simulink library "tqd"  (R2021b)
settings: Solver=VariableStepAuto  StartTime=0.0  StopTime=10.0  RelTol=1e-3
undefined symbols (not defined in the file or in its folder): ATQD_BOSEnBPSPosn_X_kph, ATQD_BOSMap_X_rpm, ATQD_BOSMap_Y_pct, ATQD_CreepBaseTqD_X_kph, ATQD_CreepBaseTqD_Y_Deg, ATQD_CreepBaseTqR_X_kph, ATQD_CreepBaseTqR_Y_Deg, ATQD_CreepBPSDisPosn_X_Deg, ATQD_CreepBPSDisPosnR_X_Deg, ATQD_CreepBPSEnPosn_X_Deg, ATQD_CreepBPSEnPosnR_X_Deg, ATQD_CreepDeltaTq_X_kph, ATQD_CreepIterm_X_kph, ATQD_CreepIterm_Y_kph, ATQD_CreepItermMaxLimit_X_pct, ATQD_CreepPreloadTime_X_kph, ATQD_CreepPreloadTq_X_kph, ATQD_CreepPreloadTq_Y_s, ATQD_CreepProtTq_X_Deg, ATQD_CreepPterm_X_kph, ATQD_ECOTqMapD_X_rpm, ATQD_ECOTqMapD_Y_pct, ATQD_NL1TqMapD_X_rpm, ATQD_NL1TqMapD_Y_pct, ATQD_NRMRrEDUSpRat_X_rpm, ATQD_NRMRrEDUSpRat_Y_Nm, ATQD_PedalMapClimbUpLim_X_rpm, ATQD_PedalMapClimbUpLim_Y_Deg, ATQD_PreLoadTq_X_s, ATQD_SL1TqMapD_X_rpm, ATQD_SL1TqMapD_Y_pct, ATQD_WhlTqCapMotGain_X_pct, ATQD_WhlTqCapMotGain_Y_mV, ENUM_ACCPEDALLOWSW_LOWIDLE, ENUM_ACCPEDALLOWSW_NOIDLE, ENUM_CHRGPLUGSTA_NONE, ENUM_CRASHSTATE_NOCRASH, ENUM_DCDCFAULTSTA_WORKING, ENUM_DRIVEMODE_ECO, ENUM_DRIVEMODE_NRM, ENUM_DRIVEMODE_SPORT, ENUM_DRIVETRAIN_AWD, ENUM_DRIVETRAIN_FWD, ENUM_DRIVETRAIN_RWD, ENUM_EBSBRKSW_PRESSED, ENUM_EBSTORQUERWQ_LIMIT, ENUM_EBSTORQUERWQ_TORQUE, ENUM_EMTRQMODE_ACCL, ENUM_EMTRQMODE_BRAKING, ENUM_EMTRQMODE_COASTING, ENUM_EPBERROR_NORMAL, ENUM_EPBSTA_APPLIED, ENUM_EPBSTA_RELEASED, ENUM_EPBSTA_UNKNOWN, ENUM_EPBSTARAW_NOTSET, ENUM_EPBSTARAW_SET, ENUM_GEARACTUALPOSN_D, ENUM_GEARACTUALPOSN_N, ENUM_GEARACTUALPOSN_P, ENUM_GEARACTUALPOSN_R ... (+201)
libraries: hcu_lib x19, simulink x12
(part 6 of 6)

== system tqd/TQD/TorqueDemand/TorqueModule/DriverWhlTqDem/RollingRegenJudge ==
  VDHP_LowIdleAccPedal_flg : Inport
  VINP_VehSpd_kph : Inport  Port=2
  VTQD_TqTargetShaftSpd_rpm : Inport  Port=3
  VTQD_RollRegenDisableReq_flg : Inport  Port=4
  VTQD_TqSourceFr_enum : Inport  Port=5
  VTQD_TqSourceRr_enum : Inport  Port=6
  VTQD_CreepEnable_flg : Inport  Port=7
  Constant : Constant  Value=ENUM_TQSOURCE_CC
  Constant1 : Constant  Value=ENUM_TQSOURCE_ADAS
  Constant2 : Constant  Value=ENUM_TQSOURCE_APS
  Constant3 : Constant  Value=ENUM_TQSOURCE_CC
  Constant4 : Constant  Value=ENUM_TQSOURCE_ADAS
  Constant5 : Constant  Value=ENUM_TQSOURCE_APS
  Detect Increase : simulink/Logic and Bit Operations/Detect Increase  vinit=0.0  OutDataTypeStr=boolean
  Equal{,1..5} (6 alike) : RelationalOperator  Operator===  OutDataTypeStr=boolean  RndMeth=Simplest
  Logical Operator : Logic  Inputs=5  AllPortsSameDT=off  OutDataTypeStr=boolean
  Logical Operator1 : Logic  Operator=NOT  AllPortsSameDT=off  OutDataTypeStr=boolean
  Logical Operator10 : Logic  Operator=OR  AllPortsSameDT=off  OutDataTypeStr=boolean
  Logical Operator11 : Logic  Operator=NOT  AllPortsSameDT=off  OutDataTypeStr=boolean
  Logical Operator12 : Logic  Operator=NOT  AllPortsSameDT=off  OutDataTypeStr=boolean
  Logical Operator5 : Logic  Operator=OR  Inputs=3  AllPortsSameDT=off  OutDataTypeStr=boolean
  Logical Operator9 : Logic  Operator=OR  Inputs=3  AllPortsSameDT=off  OutDataTypeStr=boolean
  Relay : Relay  OnSwitchValue=KTQD_RegenOnSpd_kph  OffSwitchValue=KTQD_RegenOffSpd_kph
      settings: AttributesFormatString=|
      | ON: %<OnSwitchValue>
      | OFF: %<OffSwitchValue>
  Switch2 : Switch  Criteria=u2 ~= 0
      settings: AttributesFormatString=<%<Criteria>>
  Unit Delay : UnitDelay  SampleTime=-1  HasFrameUpgradeWarning=on
  Unit Delay1 : UnitDelay  SampleTime=-1  HasFrameUpgradeWarning=on
  VTQD_RollRegenEnable_flg : Outport
  VTQD_RollingShaftSpd_rpm : Outport  Port=2
  wires:
  Equal5/1 -> Logical Operator9/3
  Equal3/1 -> Logical Operator9/1
  Equal4/1 -> Logical Operator9/2
  Constant4/1 -> Equal4/2
  [VTQD_TqSourceRr_enum] -> Equal4/1
  Constant5/1 -> Equal5/2
  [VTQD_TqSourceRr_enum] -> Equal5/1
  Constant3/1 -> Equal3/2
  [VTQD_TqSourceRr_enum] -> Equal3/1
  Constant2/1 -> Equal2/2
  [VTQD_TqSourceFr_enum] -> Equal2/1
  Constant1/1 -> Equal1/2
  [VTQD_TqSourceFr_enum] -> Equal1/1
  Constant/1 -> Equal/2
  Logical Operator11/1 -> Logical Operator/5
  Logical Operator10/1 -> Logical Operator11/1
  Logical Operator9/1 -> Logical Operator10/2
  Logical Operator5/1 -> Logical Operator10/1
  [VTQD_CreepEnable_flg] -> Unit Delay1/1
  Equal2/1 -> Logical Operator5/3
  Equal1/1 -> Logical Operator5/2
  Equal/1 -> Logical Operator5/1
  VTQD_CreepEnable_flg/1 -> [VTQD_CreepEnable_flg]
  VTQD_TqSourceFr_enum/1 -> [VTQD_TqSourceFr_enum]
  VTQD_TqSourceRr_enum/1 -> [VTQD_TqSourceRr_enum]
  [VTQD_RollRegenDisableReq_flg] -> Logical Operator1/1
  VTQD_RollRegenDisableReq_flg/1 -> [VTQD_RollRegenDisableReq_flg]
  Unit Delay/1 -> Switch2/3
  Switch2/1 -> VTQD_RollingShaftSpd_rpm/1, Unit Delay/1  "VTQD_RollingShaftSpd_rpm"
  [VTQD_TqTargetShaftSpd_rpm] -> Switch2/1
  Detect Increase/1 -> Switch2/2
  [VTQD_RollRegenEnable_flg] -> Detect Increase/1
  VTQD_TqTargetShaftSpd_rpm/1 -> [VTQD_TqTargetShaftSpd_rpm]
  [VINP_VehSpd_kph] -> Relay/1
  VINP_VehSpd_kph/1 -> [VINP_VehSpd_kph]
  VDHP_LowIdleAccPedal_flg/1 -> [VTQD_LowIdleAccPedal_flg]
  Logical Operator/1 -> VTQD_RollRegenEnable_flg/1, [VTQD_RollRegenEnable_flg]  "VTQD_RollRegenEnable_flg"
  Unit Delay1/1 -> Logical Operator12/1
  Relay/1 -> Logical Operator/2
  Logical Operator12/1 -> Logical Operator/4
  Logical Operator1/1 -> Logical Operator/3
  [VTQD_LowIdleAccPedal_flg] -> Logical Operator/1
  [VTQD_TqSourceFr_enum] -> Equal/1

== system tqd/TQD/TorqueDemand/TorqueModule/TqCoordination/Coordinate_DirverPedal ==
  VTQD_DriverWhlTqDem_Nm : Inport
  Action Port : ActionPort
  Constant9 : Constant  Value=ENUM_TQSOURCE_INTERNAL
  VTQD_DriverWhlTqReq_Nm : Outport
  VTQD_TqSourceInternal_enum : Outport  Port=2
  wires:
  VTQD_DriverWhlTqDem_Nm/1 -> VTQD_DriverWhlTqReq_Nm/1
  Constant9/1 -> VTQD_TqSourceInternal_enum/1

== system tqd/TQD/TorqueDemand/TorqueModule/TqCoordination/Coordinate_NoSuitbleGear_flg ==
  Action Port : ActionPort
  Constant5 : Constant  Value=KTQD_DriverTqDemN_Nm
  Constant8 : Constant  Value=ENUM_TQSOURCE_INVALID
  VTQD_GearNoSuitReq_Nm : Outport
  VTQD_TqSourceGearNoSuit_enum : Outport  Port=2
  wires:
  Constant5/1 -> VTQD_GearNoSuitReq_Nm/1
  Constant8/1 -> VTQD_TqSourceGearNoSuit_enum/1

== system tqd/TQD/TorqueDemand/TorqueModule/TqDistribution/AWD_Ratio ==
  VTQD_DriverWhlTqDem_Nm : Inport
  VTQD_RrShaftSpd_rpm : Inport  Port=2
  VTQD_EVDriveMode_enum : Inport  Port=3
  VTQD_LimpHomeAct_flg : Inport  Port=4
  VTQD_CreepPrLoadEnable_flg : Inport  Port=5
  Action Port : ActionPort
  Constant : Constant  Value=ONE_FLOAT
  Constant1 : Constant  Value=ONE_FLOAT
  Constant10 : Constant  Value=KTQD_AWDRrRatio_rat_ovrdflg  VectorParams1D=off  SampleTime=-1
  Constant11 : Constant  Value=KTQD_AWDRrRatio_rat_ovrdval  VectorParams1D=off  SampleTime=-1
  Constant2 : Constant  Value=ENUM_DRIVEMODE_ECO
  Constant5 : Constant  Value=ENUM_DRIVEMODE_SPORT
  Constant8 : Constant  Value=KTQD_AWDFrRatio_rat_ovrdflg  VectorParams1D=off  SampleTime=-1
  Constant9 : Constant  Value=KTQD_AWDFrRatio_rat_ovrdval  VectorParams1D=off  SampleTime=-1
  Equal : RelationalOperator  Operator===  OutDataTypeStr=boolean  RndMeth=Simplest
  Equal2 : RelationalOperator  Operator===  OutDataTypeStr=boolean  RndMeth=Simplest
  LiuzgSwitch{1..3,13} (4 alike) : Switch  Criteria=u2 ~= 0
      settings: AttributesFormatString=<%<Criteria>>
  MTQD_ECORrEDUSpRat_Z_rat : Lookup_n-D  BreakpointsForDimension1=ATQD_NRMRrEDUSpRat_Y_Nm  BreakpointsForDimension2=ATQD_NRMRrEDUSpRat_X_rpm  Table=MTQD_ECORrEDUSpRat_Z_rat  ExtrapMethod=Clip  InternalRulePriority=Speed  RndMeth=Simplest  InputSameDT=on
      settings: InputPortMap=u0,u1
  "MTQD_NRMRrEDUSpRat_Z_rat  " : Lookup_n-D  BreakpointsForDimension1=ATQD_NRMRrEDUSpRat_Y_Nm  BreakpointsForDimension2=ATQD_NRMRrEDUSpRat_X_rpm  Table=MTQD_NRMRrEDUSpRat_Z_rat  ExtrapMethod=Clip  InternalRulePriority=Speed  RndMeth=Simplest  InputSameDT=on
      settings: InputPortMap=u0,u1
  "MTQD_SPORTRrEDUSpRat_Z_rat " : Lookup_n-D  BreakpointsForDimension1=ATQD_NRMRrEDUSpRat_Y_Nm  BreakpointsForDimension2=ATQD_NRMRrEDUSpRat_X_rpm  Table=MTQD_SPORTRrEDUSpRat_Z_rat  ExtrapMethod=Clip  InternalRulePriority=Speed  RndMeth=Simplest  InputSameDT=on
      settings: InputPortMap=u0,u1
  Saturation : Saturate  UpperLimit=KTQD_RrEDUTqDistrictMax_gain  LowerLimit=KTQD_RrEDUTqDistrictMin_gain
      settings: AttributesFormatString=|
      | <%<UpperLimit>>
      | <%<LowerLimit>>
  Subtract : Sum  Inputs=+-
  Switch : Switch  Criteria=u2 > Threshold
  Switch1 : Switch  Criteria=u2 > Threshold
  VTQD_FrRatio_AWD : Outport
  VTQD_RrRatio_AWD : Outport  Port=2
  wires:
  Constant/1 -> Subtract/1
  Saturation/1 -> Switch1/3, Subtract/2
  VTQD_EVDriveMode_enum/1 -> [VTQD_EVDriveMode_enum]
  VTQD_DriverWhlTqDem_Nm/1 -> [VTQD_DriverWhlTqDem_Nm]
  VTQD_RrShaftSpd_rpm/1 -> [VTQD_RrShaftSpd_rpm]
  [VTQD_DriverWhlTqDem_Nm] -> "MTQD_NRMRrEDUSpRat_Z_rat  "/1
  [VTQD_RrShaftSpd_rpm] -> "MTQD_NRMRrEDUSpRat_Z_rat  "/2
  VTQD_LimpHomeAct_flg/1 -> [VTQD_LimpHomeAct_flg]
  [VTQD_LimpHomeAct_flg] -> LiuzgSwitch13/2
  Equal/1 -> LiuzgSwitch1/2
  "MTQD_SPORTRrEDUSpRat_Z_rat "/1 -> LiuzgSwitch1/1
  [VTQD_EVDriveMode_enum] -> Equal/1
  Constant5/1 -> Equal/2
  [VTQD_DriverWhlTqDem_Nm] -> "MTQD_SPORTRrEDUSpRat_Z_rat "/1
  [VTQD_RrShaftSpd_rpm] -> "MTQD_SPORTRrEDUSpRat_Z_rat "/2
  "MTQD_NRMRrEDUSpRat_Z_rat  "/1 -> LiuzgSwitch1/3, LiuzgSwitch13/1
  [VTQD_RrShaftSpd_rpm] -> MTQD_ECORrEDUSpRat_Z_rat/2
  [VTQD_DriverWhlTqDem_Nm] -> MTQD_ECORrEDUSpRat_Z_rat/1
  Constant2/1 -> Equal2/2
  [VTQD_EVDriveMode_enum] -> Equal2/1
  MTQD_ECORrEDUSpRat_Z_rat/1 -> LiuzgSwitch3/1
  Equal2/1 -> LiuzgSwitch3/2
  LiuzgSwitch3/1 -> LiuzgSwitch13/3
  LiuzgSwitch1/1 -> LiuzgSwitch3/3
  [VTQD_CreepPrLoadEnable_flg] -> LiuzgSwitch2/2
  Constant1/1 -> LiuzgSwitch2/1
  VTQD_CreepPrLoadEnable_flg/1 -> [VTQD_CreepPrLoadEnable_flg]
  LiuzgSwitch13/1 -> LiuzgSwitch2/3
  Subtract/1 -> Switch/3
  Switch/1 -> VTQD_FrRatio_AWD/1  "VTQD_FrEDUSpRat_rat"
  Switch1/1 -> VTQD_RrRatio_AWD/1  "VTQD_RrEDUSpRat_rat"
  Constant8/1 -> Switch/2
  Constant9/1 -> Switch/1
  Constant11/1 -> Switch1/1
  Constant10/1 -> Switch1/2
  LiuzgSwitch2/1 -> Saturation/1

== system tqd/TQD/TorqueDemand/TorqueModule/TqDistribution/FWD_Ratio ==
  Action Port : ActionPort
  Constant : Constant  Value=ONE_FLOAT
  Constant1 : Constant  Value=ZERO_FLOAT
  VTQD_FrRatio_FWD : Outport
  VTQD_RrRatio_FWD : Outport  Port=2
  wires:
  Constant/1 -> VTQD_FrRatio_FWD/1
  Constant1/1 -> VTQD_RrRatio_FWD/1

== system tqd/TQD/TorqueDemand/TorqueModule/TqDistribution/RWD_Ratio ==
  Action Port : ActionPort
  Constant : Constant  Value=ONE_FLOAT
  Constant1 : Constant  Value=ZERO_FLOAT
  VTQD_FrRatio_RWD : Outport
  VTQD_RrRatio_RWD : Outport  Port=2
  wires:
  Constant1/1 -> VTQD_FrRatio_RWD/1
  Constant/1 -> VTQD_RrRatio_RWD/1

== system tqd/TQD/TorqueDemand/TorqueModule/AvaliableTqLimit/TorqueCapacityCalcalation/CapacityDistribution ==
  VTQD_FrEDUSpRat_cmd : Inport
  VTQD_RrEDUSpRat_rat : Inport  Port=2
  VTQD_TMPwrAvailDchrg_kW : Inport  Port=3
  VINP_HVBPwrAvailChrg_kw : Inport  Port=4
  Abs1 : Abs
  Product{,1,4..5} (4 alike) : Product
  VTQD_FrHVBPwrAvailDchrg_kw : Outport
  VTQD_RrHVBPwrAvailDchrg_kw : Outport  Port=2
  VTQD_FrHVBPwrAvailChrg_kw : Outport  Port=3
  VTQD_RrHVBPwrAvailChrg_kw : Outport  Port=4
  wires:
  VTQD_RrEDUSpRat_rat/1 -> [VTQD_RrEDUSpRat_rat]
  VTQD_FrEDUSpRat_cmd/1 -> [VTQD_FrEDUSpRat_rat]
  VINP_HVBPwrAvailChrg_kw/1 -> Abs1/1
  Product4/1 -> VTQD_FrHVBPwrAvailChrg_kw/1
  Product5/1 -> VTQD_RrHVBPwrAvailChrg_kw/1
  Product1/1 -> VTQD_RrHVBPwrAvailDchrg_kw/1  "VTQD_RrHVBPwrAvailDchrg_kW"
  [VTQD_FrEDUSpRat_rat] -> Product4/1
  [VTQD_FrEDUSpRat_rat] -> Product/1
  Abs1/1 -> Product4/2, Product5/1
  VTQD_TMPwrAvailDchrg_kW/1 -> Product1/1, Product/2
  [VTQD_RrEDUSpRat_rat] -> Product5/2
  Product/1 -> VTQD_FrHVBPwrAvailDchrg_kw/1  "VTQD_FrHVBPwrAvailDchrg_kW"
  [VTQD_RrEDUSpRat_rat] -> Product1/2

== system tqd/TQD/TorqueDemand/TorqueModule/AvaliableTqLimit/TorqueCapacityCalcalation/Generation ==
  VTQD_FrShaftSpd_rpm : Inport
  VTQD_RrShaftSpd_rpm : Inport  Port=2
  VTQD_FrHVBPwrAvailChrg_kw : Inport  Port=3
  VTQD_RrHVBPwrAvailChrg_kw : Inport  Port=4
  KTQD_FrBatapCont_factor : Inport  Port=5
  KTQD_RrBatapCont_factor : Inport  Port=6
  Abs2 : Abs
  Abs6 : Abs
  Constant : Constant  Value=KTQD_WhlTqCap_ovrdflg
  Constant1 : Constant  Value=KTQD_WhlTqCapGen_ovrdval
  Constant2 : Constant  Value=KTQD_RrTMSpdMin_rpm  OutDataTypeStr=single
  Constant3 : Constant  Value=KTQD_WhlTqCap_ovrdflg
  Constant5 : Constant  Value=KTQD_FrTMSpdMin_rpm  OutDataTypeStr=single
  Constant7 : Constant  Value=KTQD_WhlTqCapGen_ovrdval
  Fcn : Fcn  Expr=u[1]/u[2]/pi*u[3]
  Fcn2 : Fcn  Expr=u[1]/u[2]/pi*u[3]
  Gain1 : Gain  Gain=-1
  Gain4 : Gain  Gain=-1
  Max1 : MinMax  Function=max  Inputs=2
  Max4 : MinMax  Function=max  Inputs=2
  Mux : Mux  Inputs=3
  Mux2 : Mux  Inputs=3
  Saturation1 : Saturate  UpperLimit=0  LowerLimit=KTQD_FrLowTheldTrq_Nm
      settings: AttributesFormatString=|
      | Upper Limit :%<UpperLimit>
      | Lower Limit :%<LowerLimit>
  Saturation2 : Saturate  UpperLimit=0  LowerLimit=KTQD_RrLowTheldTrq_Nm
      settings: AttributesFormatString=|
      | Upper Limit :%<UpperLimit>
      | Lower Limit :%<LowerLimit>
  Switch : Switch  Criteria=u2 ~= 0
      settings: AttributesFormatString=<%<Criteria>>
  Switch1 : Switch  Criteria=u2 ~= 0
      settings: AttributesFormatString=<%<Criteria>>
  VTQD_WhlTqCapGenFr_Nm : Outport
  VTQD_WhlTqCapGenRr_Nm : Outport  Port=2
  wires:
  Gain1/1 -> Saturation2/1
  Gain4/1 -> Saturation1/1
  Saturation2/1 -> Switch1/3
  Switch1/1 -> VTQD_WhlTqCapGenRr_Nm/1  "VTQD_WhlTqCapGenRr_Nm"
  Constant3/1 -> Switch1/2
  Constant7/1 -> Switch1/1
  Saturation1/1 -> Switch/3
  Switch/1 -> VTQD_WhlTqCapGenFr_Nm/1  "VTQD_WhlTqCapGenFr_Nm"
  Constant1/1 -> Switch/1
  Constant/1 -> Switch/2
  VTQD_RrHVBPwrAvailChrg_kw/1 -> [VTQD_RrHVBPwrAvailChrg_kw]
  KTQD_FrBatapCont_factor/1 -> [KTQD_FrBatapCont_factor]
  VTQD_FrHVBPwrAvailChrg_kw/1 -> [VTQD_FrHVBPwrAvailChrg_kw]
  VTQD_FrShaftSpd_rpm/1 -> [VTQD_FrShaftSpd_rpm]
  VTQD_RrShaftSpd_rpm/1 -> [VTQD_RrShaftSpd_rpm]
  KTQD_RrBatapCont_factor/1 -> [KTQD_RrBatapCont_factor]
  Fcn2/1 -> Gain1/1
  Max1/1 -> Mux2/2
  Abs2/1 -> Max1/1
  Mux2/1 -> Fcn2/1
  Constant2/1 -> Max1/2
  [KTQD_RrBatapCont_factor] -> Mux2/3
  [VTQD_RrShaftSpd_rpm] -> Abs2/1
  [VTQD_RrHVBPwrAvailChrg_kw] -> Mux2/1
  Fcn/1 -> Gain4/1
  Abs6/1 -> Max4/1
  [VTQD_FrHVBPwrAvailChrg_kw] -> Mux/1
  Constant5/1 -> Max4/2
  [VTQD_FrShaftSpd_rpm] -> Abs6/1
  [KTQD_FrBatapCont_factor] -> Mux/3
  Mux/1 -> Fcn/1
  Max4/1 -> Mux/2

== system tqd/TQD/TorqueDemand/TorqueModule/AvaliableTqLimit/TorqueCapacityCalcalation/Motoring ==
  VTQD_FrShaftSpd_rpm : Inport
  VTQD_RrShaftSpd_rpm : Inport  Port=2
  VTQD_FrHVBPwrAvailDchrg_kw : Inport  Port=3
  VTQD_RrHVBPwrAvailDchrg_kw : Inport  Port=4
  KTQD_FrBatapCont_factor : Inport  Port=5
  KTQD_RrBatapCont_factor : Inport  Port=6
  VINP_HVBCellVoltMax_mV : Inport  Port=7
  VINP_HVBCellVoltMin_mV : Inport  Port=8
  VINP_HVBSOH_pct : Inport  Port=9
  Abs : Abs
  Abs2 : Abs
  Add : Sum  Commented=on  Inputs=+-
  Constant : Constant  Value=KTQD_WhlTqCap_ovrdflg
  Constant1 : Constant  Value=KTQD_FrTMSpdMin_rpm  OutDataTypeStr=single
  Constant2 : Constant  Value=ZERO_FLOAT
  Constant3 : Constant  Value=KTQD_RrTMSpdMin_rpm  OutDataTypeStr=single
  Constant4 : Constant  Value=ZERO_FLOAT
  Constant5 : Constant  Value=KTQD_WhlTqCapMot_ovrdval
  Constant6 : Constant  Value=KTQD_WhlTqCap_ovrdflg
  Constant7 : Constant  Value=KTQD_WhlTqCapMot_ovrdval
  Constant8 : Constant  Value=KTQD_FrUppTheldTrq_Nm
  Constant9 : Constant  Value=KTQD_RrUppTheldTrq_Nm
  Fcn : Fcn  Expr=u[1]/u[2]/pi*u[3]
  Fcn2 : Fcn  Expr=u[1]/u[2]/pi*u[3]
  From3 : From  Commented=on  GotoTag=VINP_HVBCellVoltMax_mV
  From4 : From  Commented=on  GotoTag=VINP_HVBCellVoltMin_mV
  From5 : From  Commented=on  GotoTag=VTQD_HCBCellVoltDev_mV
  From6 : From  Commented=on  GotoTag=VINP_HVBSOH_pct
  Goto7 : Goto  Commented=on  GotoTag=VTQD_HCBCellVoltDev_mV
  Goto9 : Goto  Commented=on  GotoTag=VTQD_WhlTqCapMotGain_c
  MTQD_WhlTqCapMotGain_Z_c : Lookup_n-D  Commented=on  BreakpointsForDimension1=ATQD_WhlTqCapMotGain_Y_mV  BreakpointsForDimension2=ATQD_WhlTqCapMotGain_X_pct  Table=MTQD_WhlTqCapMotGain_Z_c  InternalRulePriority=Speed  RndMeth=Simplest  InputSameDT=on
      settings: InputPortMap=u0,u1
  Max{,1..3} (4 alike) : MinMax  Function=max  Inputs=2
  Min : MinMax  Inputs=2
  Min1 : MinMax  Inputs=2
  Mux : Mux  Inputs=3
  Mux2 : Mux  Inputs=3
  Switch : Switch  Criteria=u2 ~= 0
      settings: AttributesFormatString=<%<Criteria>>
  Switch1 : Switch  Criteria=u2 ~= 0
      settings: AttributesFormatString=<%<Criteria>>
  Terminator : Terminator
  Terminator1 : Terminator
  Terminator2 : Terminator
  VTQD_WhlTqCapMotFr_Nm : Outport
  VTQD_WhlTqCapMotRr_Nm : Outport  Port=2
  wires:
  Fcn2/1 -> Min1/1
  Switch1/1 -> VTQD_WhlTqCapMotRr_Nm/1  "VTQD_WhlTqCapMotRr_Nm"
  Constant7/1 -> Switch1/1
  Constant6/1 -> Switch1/2
  Constant5/1 -> Switch/1
  Constant/1 -> Switch/2
  Switch/1 -> VTQD_WhlTqCapMotFr_Nm/1  "VTQD_WhlTqCapMotFr_Nm"
  VTQD_RrHVBPwrAvailDchrg_kw/1 -> [VTQD_RrHVBPwrAvailDchrg_kw]
  KTQD_RrBatapCont_factor/1 -> [KTQD_RrBatapCont_factor]
  VTQD_RrShaftSpd_rpm/1 -> [VTQD_RrShaftSpd_rpm]
  Abs2/1 -> Max2/1
  [VTQD_RrHVBPwrAvailDchrg_kw] -> Mux2/1
  Constant3/1 -> Max2/2
  [VTQD_RrShaftSpd_rpm] -> Abs2/1
  Mux2/1 -> Fcn2/1
  Max2/1 -> Mux2/2
  [VTQD_FrHVBPwrAvailDchrg_kw] -> Mux/1
  Max/1 -> Mux/2
  [VTQD_FrShaftSpd_rpm] -> Abs/1
  KTQD_FrBatapCont_factor/1 -> [KTQD_FrBatapCont_factor]
  VTQD_FrHVBPwrAvailDchrg_kw/1 -> [VTQD_FrHVBPwrAvailDchrg_kw]
  Abs/1 -> Max/1
  Fcn/1 -> Min/1
  Mux/1 -> Fcn/1
  VTQD_FrShaftSpd_rpm/1 -> [VTQD_FrShaftSpd_rpm]
  Constant1/1 -> Max/2
  Constant8/1 -> Min/2
  Min/1 -> Max1/1
  Constant2/1 -> Max1/2
  Constant9/1 -> Min1/2
  Min1/1 -> Max3/1
  Constant4/1 -> Max3/2
  VINP_HVBCellVoltMin_mV/1 -> Terminator1/1
  VINP_HVBSOH_pct/1 -> Terminator2/1
  VINP_HVBCellVoltMax_mV/1 -> Terminator/1
  Add/1 -> Goto7/1  "VTQD_HCBCellVoltDev_mV"
  From3/1 -> Add/1
  From4/1 -> Add/2
  From5/1 -> MTQD_WhlTqCapMotGain_Z_c/1
  [KTQD_FrBatapCont_factor] -> Mux/3
  [KTQD_RrBatapCont_factor] -> Mux2/3
  MTQD_WhlTqCapMotGain_Z_c/1 -> Goto9/1  "VTQD_WhlTqCapMotGain_c"
  Max1/1 -> Switch/3
  Max3/1 -> Switch1/3
  From6/1 -> MTQD_WhlTqCapMotGain_Z_c/2

== system tqd/TQD/TorqueDemand/TorqueModule/AvaliableTqLimit/TorqueCapacityCalcalation/TMAvailablePwr_Calculation ==
  VINP_HVBPwrAvailDchrg_kw : Inport
  Add : Sum
  Constant : Constant  Value=KTQD_DCDCCalPwrAvailRsv_kW
  Constant1 : Constant  Value=KTQD_THCMCalPwrAvailRsv_kW
  Constant2 : Constant  Value=KTQD_TMPwrAvailDchrg_kW_ovrdflg
  Constant3 : Constant  Value=ZERO_FLOAT
  Min : MinMax  Function=max  Inputs=2
  Subtract : Sum  Inputs=+-
  Switch : Switch  Criteria=u2 ~= 0
      settings: AttributesFormatString=<%<Criteria>>
  VTQD_TMPwrAvailDchrg_kW : Outport
  wires:
  Constant3/1 -> Min/2
  Min/1 -> Switch/1
  Switch/1 -> VTQD_TMPwrAvailDchrg_kW/1  "VTQD_TMPwrAvailDchrg_kW"
  Constant2/1 -> Switch/2
  Subtract/1 -> Min/1
  Add/1 -> Subtract/2
  VINP_HVBPwrAvailDchrg_kw/1 -> Subtract/1, Switch/3
  Constant1/1 -> Add/2
  Constant/1 -> Add/1

== system tqd/TQD/TorqueDemand/TorqueModule/DriverWhlTqDem/Creep/If Action Subsystem ==
  In1 : Inport
  Action Port : ActionPort
  Out1 : Outport
  wires:
  In1/1 -> Out1/1

== system tqd/TQD/TorqueDemand/TorqueModule/DriverWhlTqDem/Creep/If Action Subsystem1 ==
  VTQD_ActBPSPosnInRange_flg : Inport
  VTQD_CreepErrSpd_kph : Inport  Port=2
  VTQD_CreepPterm_c : Inport  Port=3
  VTQD_CreepIterm_c : Inport  Port=4
  VTQD_CreepDeltaTq_Nm : Inport  Port=5
  VTQD_ActBPSPosn_pct : Inport  Port=6
  task_time_s : Inport  Port=7
  VTQD_CreepDisable_flg : Inport  Port=8
  VTQD_CreepEnable_flg : Inport  Port=9
  VTQD_OPDOn2Off : Inport  Port=10
  Add : Sum
  Add1 : Sum  Inputs=+++
  Constant : Constant  Value=ZERO_FLOAT
  Constant1 : Constant  Value=KTQD_CreepItermMinLimit_Nm
  Constant4 : Constant  Value=ZERO_FLOAT
  Constant5 : Constant  Value=ONE_FLOAT
  Data Type Conversion : DataTypeConversion
  Goto1 : Goto  Commented=on  GotoTag=VTQD_CreepErrSpd_kph
  Goto6 : Goto  Commented=on  GotoTag=task_time_s
  Ground1 : Ground  Commented=on
  Ground6 : Ground  Commented=on
  MTQD_CreepItermMaxLimit_Y_Nm : Lookup_n-D  NumberOfTableDimensions=1  BreakpointsForDimension1=ATQD_CreepItermMaxLimit_X_pct  Table=MTQD_CreepItermMaxLimit_Y_Nm  ExtrapMethod=Clip  InternalRulePriority=Speed  RndMeth=Simplest  InputSameDT=on
  NOT : Logic  Operator=NOT  AllPortsSameDT=off  OutDataTypeStr=boolean
  OR : Logic  Operator=OR  Inputs=4  AllPortsSameDT=off  OutDataTypeStr=boolean
  Product : Product
  Product2 : Product
  Saturation Dynamic : simulink/Discontinuities/Saturation Dynamic  OutMin=[]  OutMax=[]  OutDataTypeStr=Inherit: Same as second input  OutDataType=fixdt(1, 16)  OutScaling=2^-10  DoSatur=off
  Switch1 : Switch  Criteria=u2 ~= 0
  Switch4 : Switch  Criteria=u2 ~= 0
  Terminator1 : Terminator
  Terminator2 : Terminator
  Unit Delay : UnitDelay  SampleTime=-1  HasFrameUpgradeWarning=on
  VTQD_CreepTotalOfstTq_Nm : Outport
  wires:
  Add1/1 -> VTQD_CreepTotalOfstTq_Nm/1  "VTQD_CreepTotalOfstTq_Nm"
  VTQD_CreepDeltaTq_Nm/1 -> [VTQD_CreepDeltaTq_Nm]
  VTQD_CreepIterm_c/1 -> [VTQD_CreepIterm_c]
  VTQD_CreepPterm_c/1 -> [VTQD_CreepPterm_c]
  VTQD_ActBPSPosnInRange_flg/1 -> [VTQD_ActBPSPosnInRange_flg]
  task_time_s/1 -> Terminator1/1
  VTQD_ActBPSPosn_pct/1 -> [VTQD_ActBPSPosn_pct]
  Ground1/1 -> Goto6/1
  VTQD_CreepErrSpd_kph/1 -> Terminator2/1
  Ground6/1 -> Goto1/1
  VTQD_CreepDisable_flg/1 -> [VTQD_CreepDisable_flg]
  OR/1 -> [VTQD_CreepPICtrlReset_flg]  "VTQD_CreepPICtrlReset_flg"
  VTQD_CreepEnable_flg/1 -> [VTQD_CreepEnable_flg]
  VTQD_OPDOn2Off/1 -> [VTQD_OPDOn2Off_flg]
  [VTQD_OPDOn2Off_flg] -> OR/2
  [VTQD_CreepDisable_flg] -> OR/3
  [VTQD_ActBPSPosnInRange_flg] -> OR/1
  [VTQD_CreepEnable_flg] -> NOT/1
  NOT/1 -> OR/4
  Data Type Conversion/1 -> Add1/3  "VTQD_CreepOffsetTq_Nm"
  Constant1/1 -> Saturation Dynamic/3
  [VTQD_ActBPSPosn_pct] -> MTQD_CreepItermMaxLimit_Y_Nm/1
  [VTQD_CreepPICtrlReset_flg] -> Switch4/2
  MTQD_CreepItermMaxLimit_Y_Nm/1 -> Saturation Dynamic/1  "VTQD_CreepItermMaxLimit_Nm"
  Constant/1 -> Switch1/1
  Product/1 -> Switch1/3
  [VTQD_CreepPterm_c] -> Product/1
  Constant5/1 -> Product/2, Product2/1
  [VTQD_CreepPICtrlReset_flg] -> Switch1/2
  Add/1 -> Switch4/3
  Switch1/1 -> Add1/1  "VTQD_CreepPtermTq_Nm"
  Saturation Dynamic/1 -> Add1/2  "VTQD_CreepItermTq_Nm"
  Product2/1 -> Add/1
  Switch4/1 -> Unit Delay/1, Saturation Dynamic/2
  Unit Delay/1 -> Add/2
  Constant4/1 -> Switch4/1
  [VTQD_CreepIterm_c] -> Product2/2
  [VTQD_CreepDeltaTq_Nm] -> Data Type Conversion/1

== system tqd/TQD/TorqueDemand/TorqueModule/DriverWhlTqDem/Creep/Switch Case Action Subsystem ==
  In1 : Inport
  Action Port : ActionPort
  Out1 : Outport
  wires:
  In1/1 -> Out1/1

== system tqd/TQD/TorqueDemand/TorqueModule/DriverWhlTqDem/PedalMapWhlTq/LHM ==
  VTQD_ActAPSPosn_pct : Inport
  VTQD_TqTargetShaftSpd_rpm : Inport  Port=2
  VTQD_GearActualPosn_enum : Inport  Port=3
  Action Port : ActionPort
  Constant : Constant  Value=ZERO_FLOAT
  Constant1 : Constant  Value=ENUM_GEARACTUALPOSN_D
  Constant2 : Constant  Value=ENUM_GEARACTUALPOSN_R
  Equal1 : RelationalOperator  Operator===  OutDataTypeStr=boolean  RndMeth=Simplest
  Equal2 : RelationalOperator  Operator===  OutDataTypeStr=boolean  RndMeth=Simplest
  MTQD_LHMTqMapD_Z_Nm : Lookup_n-D  BreakpointsForDimension1=ATQD_NL1TqMapD_Y_pct  BreakpointsForDimension2=ATQD_NL1TqMapD_X_rpm  Table=MTQD_LHMTqMapD_Z_Nm  ExtrapMethod=Clip  InternalRulePriority=Speed  RndMeth=Simplest  InputSameDT=on
      settings: InputPortMap=u0,u1
  MTQD_LHMTqMapR_Z_Nm : Lookup_n-D  BreakpointsForDimension1=ATQD_NL1TqMapD_Y_pct  BreakpointsForDimension2=ATQD_NL1TqMapD_X_rpm  Table=MTQD_LHMTqMapR_Z_Nm  ExtrapMethod=Clip  InternalRulePriority=Speed  RndMeth=Simplest  InputSameDT=on
      settings: InputPortMap=u0,u1
  Switch1 : Switch  Criteria=u2 ~= 0
  Switch2 : Switch  Criteria=u2 ~= 0
  VTQD_PedalMapWhlTqLHM_Nm : Outport
  wires:
  Switch1/1 -> VTQD_PedalMapWhlTqLHM_Nm/1
  Constant/1 -> Switch2/3
  [VTQD_LHMTqMapR_Nm] -> Switch2/1
  Equal2/1 -> Switch2/2
  Constant2/1 -> Equal2/2
  [VTQD_GearActualPosn_enum] -> Equal2/1
  Switch2/1 -> Switch1/3
  [VTQD_LHMTqMapD_Nm] -> Switch1/1
  Constant1/1 -> Equal1/2
  Equal1/1 -> Switch1/2
  [VTQD_GearActualPosn_enum] -> Equal1/1
  [VTQD_TqTargetShaftSpd_rpm] -> MTQD_LHMTqMapR_Z_Nm/2
  [VTQD_ActAPSPosn_pct] -> MTQD_LHMTqMapR_Z_Nm/1
  MTQD_LHMTqMapR_Z_Nm/1 -> [VTQD_LHMTqMapR_Nm]
  MTQD_LHMTqMapD_Z_Nm/1 -> [VTQD_LHMTqMapD_Nm]
  [VTQD_TqTargetShaftSpd_rpm] -> MTQD_LHMTqMapD_Z_Nm/2
  [VTQD_ActAPSPosn_pct] -> MTQD_LHMTqMapD_Z_Nm/1
  VTQD_GearActualPosn_enum/1 -> [VTQD_GearActualPosn_enum]
  VTQD_TqTargetShaftSpd_rpm/1 -> [VTQD_TqTargetShaftSpd_rpm]
  VTQD_ActAPSPosn_pct/1 -> [VTQD_ActAPSPosn_pct]

== system tqd/TQD/TorqueDemand/TorqueModule/DriverWhlTqDem/PedalMapWhlTq/NoLHM ==
  VTQD_ActAPSPosn_pct : Inport
  VTQD_TqTargetShaftSpd_rpm : Inport  Port=2
  VTQD_RegenMode_enum : Inport  Port=3
  VTQD_GearActualPosn_enum : Inport  Port=4
  VTQD_EVDriveMode_enum : Inport  Port=5
  Action Port : ActionPort
  Constant11 : Constant  Value=ENUM_GEARACTUALPOSN_D
  Constant12 : Constant  Value=ENUM_GEARACTUALPOSN_R
  Equal7 : RelationalOperator  Operator===  OutDataTypeStr=boolean  RndMeth=Simplest
  Equal8 : RelationalOperator  Operator===  OutDataTypeStr=boolean  RndMeth=Simplest
  GearShiftCheck : If  NumInputs=2  IfExpression=u1~= 0  ElseIfExpressions=u2~= 0
  Merge1 : Merge  Inputs=3
  ShiftD : Subsystem  TreatAsAtomicUnit=on
  ShiftPorN : Subsystem  TreatAsAtomicUnit=on
  ShiftR : Subsystem  TreatAsAtomicUnit=on
  VTQD_PedalMapWhlTqNoLHM_Nm : Outport
  wires:
  ShiftR/1(VTQD_PedalMapWhlTqR_Nm) -> Merge1/2
  VTQD_EVDriveMode_enum/1 -> [VTQD_EVDriveMode_enum]
  VTQD_GearActualPosn_enum/1 -> [VTQD_GearActualPosn_enum]
  [VTQD_TqTargetShaftSpd_rpm] -> ShiftD/3(VTQD_TqTargetShaftSpd_rpm)
  Equal7/1 -> GearShiftCheck/1
  GearShiftCheck/3 -> ShiftPorN/Action
  Equal8/1 -> GearShiftCheck/2
  [VTQD_ActAPSPosn_pct] -> ShiftR/1(VTQD_ActAPSPosn_pct)
  ShiftPorN/1(VTQD_PedalMapWhlTqPorN_Nm) -> Merge1/3
  [VTQD_EVDriveMode_enum] -> ShiftD/1(VTQD_EVDriveMode_enum)
  [VTQD_TqTargetShaftSpd_rpm] -> ShiftR/2(VTQD_TqTargetShaftSpd_rpm)
  GearShiftCheck/1 -> ShiftD/Action
  Merge1/1 -> VTQD_PedalMapWhlTqNoLHM_Nm/1  "VTQD_PedalMapWhlTqNoLHM_Nm"
  Constant12/1 -> Equal8/2
  Constant11/1 -> Equal7/2
  GearShiftCheck/2 -> ShiftR/Action
  [VTQD_GearActualPosn_enum] -> Equal7/1
  [VTQD_ActAPSPosn_pct] -> ShiftD/2(VTQD_ActAPSPosn_pct)
  [VTQD_GearActualPosn_enum] -> Equal8/1
  ShiftD/1(VTQD_PedalMapWhlTqD_Nm) -> Merge1/1
  VTQD_RegenMode_enum/1 -> [VTQD_RegenMode_enum]
  VTQD_ActAPSPosn_pct/1 -> [VTQD_ActAPSPosn_pct]
  VTQD_TqTargetShaftSpd_rpm/1 -> [VTQD_TqTargetShaftSpd_rpm]
  [VTQD_RegenMode_enum] -> ShiftD/4(VTQD_RegenMode_enum)

== system tqd/TQD/TorqueDemand/TorqueModule/DriverWhlTqDem/PedalMapWhlTq/NoLHM/ShiftD ==
  VTQD_EVDriveMode_enum : Inport
  VTQD_ActAPSPosn_pct : Inport  Port=2
  VTQD_TqTargetShaftSpd_rpm : Inport  Port=3
  VTQD_RegenMode_enum : Inport  Port=4
  Action Port : ActionPort
  Constant5 : Constant  Value=ENUM_DRIVEMODE_NRM
  Constant6 : Constant  Value=ENUM_DRIVEMODE_ECO
  Constant7 : Constant  Value=ENUM_DRIVEMODE_SPORT
  Equal1 : RelationalOperator  Operator===  OutDataTypeStr=boolean  RndMeth=Simplest
  Equal2 : RelationalOperator  Operator===  OutDataTypeStr=boolean  RndMeth=Simplest
  Equal3 : RelationalOperator  Operator===  OutDataTypeStr=boolean  RndMeth=Simplest
  If : If  NumInputs=3  IfExpression=u1 ~= 0  ElseIfExpressions=u2 ~= 0
  LUT_D_ECO : Subsystem  TreatAsAtomicUnit=on
  LUT_D_Normal : Subsystem  TreatAsAtomicUnit=on
  LUT_D_Sport : Subsystem  TreatAsAtomicUnit=on
  Merge : Merge  Inputs=3
  VTQD_PedalMapWhlTqD_Nm : Outport
  wires:
  [VTQD_TqTargetShaftSpd_rpm] -> LUT_D_Sport/1(VTQD_TqTargetShaftSpd_rpm)
  [VTQD_ActAPSPosn_pct] -> LUT_D_Sport/2(VTQD_ActAPSPosn_pct)
  [VTQD_RegenMode_enum] -> LUT_D_Sport/3(VTQD_RegenMode_enum)
  [VTQD_ActAPSPosn_pct] -> LUT_D_ECO/2(VTQD_ActAPSPosn_pct)
  [VTQD_TqTargetShaftSpd_rpm] -> LUT_D_ECO/1(VTQD_TqTargetShaftSpd_rpm)
  LUT_D_Normal/1(VTQD_WhlTqNRMD_Nm) -> Merge/1
  If/3 -> LUT_D_Sport/Action
  If/2 -> LUT_D_ECO/Action
  If/1 -> LUT_D_Normal/Action
  LUT_D_ECO/1(VTQD_WhlTqECOD_Nm) -> Merge/2
  LUT_D_Sport/1(VTQD_WhlTqSPORTD_Nm) -> Merge/3
  Equal3/1 -> If/3
  Equal2/1 -> If/2
  Equal1/1 -> If/1
  [VTQD_ActAPSPosn_pct] -> LUT_D_Normal/2(VTQD_ActAPSPosn_pct)
  [VTQD_TqTargetShaftSpd_rpm] -> LUT_D_Normal/1(VTQD_TqTargetShaftSpd_rpm)
  [VTQD_RegenMode_enum] -> LUT_D_Normal/3(VTQD_RegenMode_enum)
  VTQD_RegenMode_enum/1 -> [VTQD_RegenMode_enum]
  VTQD_TqTargetShaftSpd_rpm/1 -> [VTQD_TqTargetShaftSpd_rpm]
  VTQD_ActAPSPosn_pct/1 -> [VTQD_ActAPSPosn_pct]
  VTQD_EVDriveMode_enum/1 -> [VTQD_EVDriveMode_enum]
  Merge/1 -> VTQD_PedalMapWhlTqD_Nm/1
  Constant7/1 -> Equal3/2
  Constant5/1 -> Equal1/2
  [VTQD_EVDriveMode_enum] -> Equal3/1
  Constant6/1 -> Equal2/2
  [VTQD_EVDriveMode_enum] -> Equal2/1
  [VTQD_EVDriveMode_enum] -> Equal1/1
  [VTQD_RegenMode_enum] -> LUT_D_ECO/3(VTQD_RegenMode_enum)

== system tqd/TQD/TorqueDemand/TorqueModule/DriverWhlTqDem/PedalMapWhlTq/NoLHM/ShiftPorN ==
  Action Port : ActionPort
  Constant : Constant  Value=ZERO_FLOAT
  VTQD_PedalMapWhlTqPorN_Nm : Outport
  wires:
  Constant/1 -> VTQD_PedalMapWhlTqPorN_Nm/1

== system tqd/TQD/TorqueDemand/TorqueModule/DriverWhlTqDem/PedalMapWhlTq/NoLHM/ShiftR ==
  VTQD_ActAPSPosn_pct : Inport
  VTQD_TqTargetShaftSpd_rpm : Inport  Port=2
  Action Port : ActionPort
  MTQD_NRMTqMapR_Z_Nm : Lookup_n-D  BreakpointsForDimension1=ATQD_NL1TqMapD_Y_pct  BreakpointsForDimension2=ATQD_NL1TqMapD_X_rpm  Table=MTQD_NRMTqMapR_Z_Nm  ExtrapMethod=Clip  InternalRulePriority=Speed  RndMeth=Simplest  InputSameDT=on
      settings: InputPortMap=u0,u1
  VTQD_PedalMapWhlTqR_Nm : Outport
  wires:
  [VTQD_NRMTqMapR_Nm] -> VTQD_PedalMapWhlTqR_Nm/1
  MTQD_NRMTqMapR_Z_Nm/1 -> [VTQD_NRMTqMapR_Nm]
  [VTQD_ActAPSPosn_pct] -> MTQD_NRMTqMapR_Z_Nm/1
  [VTQD_TqTargetShaftSpd_rpm] -> MTQD_NRMTqMapR_Z_Nm/2
  VTQD_ActAPSPosn_pct/1 -> [VTQD_ActAPSPosn_pct]
  VTQD_TqTargetShaftSpd_rpm/1 -> [VTQD_TqTargetShaftSpd_rpm]

== system tqd/TQD/TorqueDemand/TorqueModule/DriverWhlTqDem/PedalMapWhlTq/NoLHM/ShiftD/LUT_D_ECO ==
  VTQD_TqTargetShaftSpd_rpm : Inport
  VTQD_ActAPSPosn_pct : Inport  Port=2
  VTQD_RegenMode_enum : Inport  Port=3
  Action Port : ActionPort
  MTQD_ECOTqMapD_Z_Nm : Lookup_n-D  BreakpointsForDimension1=ATQD_ECOTqMapD_Y_pct  BreakpointsForDimension2=ATQD_ECOTqMapD_X_rpm  Table=MTQD_ECOTqMapD_Z_Nm  ExtrapMethod=Clip  InternalRulePriority=Speed  RndMeth=Simplest  InputSameDT=on
      settings: InputPortMap=u0,u1
  Terminator : Terminator
  VTQD_WhlTqECOD_Nm : Outport
  wires:
  [VTQD_ActAPSPosn_pct] -> MTQD_ECOTqMapD_Z_Nm/1
  [VTQD_TqTargetShaftSpd_rpm] -> MTQD_ECOTqMapD_Z_Nm/2
  VTQD_ActAPSPosn_pct/1 -> [VTQD_ActAPSPosn_pct]
  VTQD_TqTargetShaftSpd_rpm/1 -> [VTQD_TqTargetShaftSpd_rpm]
  MTQD_ECOTqMapD_Z_Nm/1 -> [VTQD_ECOTqMapD_Nm]
  [VTQD_ECOTqMapD_Nm] -> VTQD_WhlTqECOD_Nm/1
  VTQD_RegenMode_enum/1 -> Terminator/1

== system tqd/TQD/TorqueDemand/TorqueModule/DriverWhlTqDem/PedalMapWhlTq/NoLHM/ShiftD/LUT_D_Normal ==
  VTQD_TqTargetShaftSpd_rpm : Inport
  VTQD_ActAPSPosn_pct : Inport  Port=2
  VTQD_RegenMode_enum : Inport  Port=3
  Action Port : ActionPort
  MTQD_NL1TqMapD_Z_Nm : Lookup_n-D  BreakpointsForDimension1=ATQD_NL1TqMapD_Y_pct  BreakpointsForDimension2=ATQD_NL1TqMapD_X_rpm  Table=MTQD_NL1TqMapD_Z_Nm  ExtrapMethod=Clip  InternalRulePriority=Speed  RndMeth=Simplest  InputSameDT=on
      settings: InputPortMap=u0,u1
  Terminator : Terminator
  VTQD_WhlTqNRMD_Nm : Outport
  wires:
  [VTQD_NL1TqMapD_Nm] -> VTQD_WhlTqNRMD_Nm/1
  [VTQD_ActAPSPosn_pct] -> MTQD_NL1TqMapD_Z_Nm/1
  [VTQD_TqTargetShaftSpd_rpm] -> MTQD_NL1TqMapD_Z_Nm/2
  VTQD_RegenMode_enum/1 -> Terminator/1
  VTQD_ActAPSPosn_pct/1 -> [VTQD_ActAPSPosn_pct]
  VTQD_TqTargetShaftSpd_rpm/1 -> [VTQD_TqTargetShaftSpd_rpm]
  MTQD_NL1TqMapD_Z_Nm/1 -> [VTQD_NL1TqMapD_Nm]

== system tqd/TQD/TorqueDemand/TorqueModule/DriverWhlTqDem/PedalMapWhlTq/NoLHM/ShiftD/LUT_D_Sport ==
  VTQD_TqTargetShaftSpd_rpm : Inport
  VTQD_ActAPSPosn_pct : Inport  Port=2
  VTQD_RegenMode_enum : Inport  Port=3
  Action Port : ActionPort
  MTQD_SL1TqMapD_Z_Nm : Lookup_n-D  BreakpointsForDimension1=ATQD_SL1TqMapD_Y_pct  BreakpointsForDimension2=ATQD_SL1TqMapD_X_rpm  Table=MTQD_SL1TqMapD_Z_Nm  ExtrapMethod=Clip  InternalRulePriority=Speed  RndMeth=Simplest  InputSameDT=on
      settings: InputPortMap=u0,u1
  Terminator : Terminator
  VTQD_WhlTqSPORTD_Nm : Outport
  wires:
  [VTQD_SL1TqMapD_Nm] -> VTQD_WhlTqSPORTD_Nm/1
  [VTQD_ActAPSPosn_pct] -> MTQD_SL1TqMapD_Z_Nm/1
  [VTQD_TqTargetShaftSpd_rpm] -> MTQD_SL1TqMapD_Z_Nm/2
  VTQD_RegenMode_enum/1 -> Terminator/1
  VTQD_ActAPSPosn_pct/1 -> [VTQD_ActAPSPosn_pct]
  VTQD_TqTargetShaftSpd_rpm/1 -> [VTQD_TqTargetShaftSpd_rpm]
  MTQD_SL1TqMapD_Z_Nm/1 -> [VTQD_SL1TqMapD_Nm]

== stateflow chart tqd/TQD/TorqueDemand/ShiftModule/Determine_Actual_Gear_Position ==
  state Initialize [commented out]
    en:
    VTQD_GearActualPosn_enum = ENUM_GEARACTUALPOSN_INVALID;
    VTQD_ShiftInitialComplete_flg = FALSE;
    (default) -> (junction 489) [commented out] : {
        | VTQD_InitializeTime_s = 0;
        | }
    Initialize -> (junction 489) [commented out]
    (junction 489) -> (junction 490) [commented out] : [VTQD_InitializeTime_s > KTQD_ShiftInitialTime_s]
    (junction 489) -> (junction 531) [commented out] : {
        | VTQD_InitializeTime_s = VTQD_InitializeTime_s + task_time_s;
        | }
    (junction 490) -> (junction 533) [commented out] : {
        | VTQD_ShiftInitialComplete_flg = TRUE;
        | }
    (junction 533) -> (junction 531) [commented out]
  state PBW_Judgement [commented out]
    en:
    VTQD_PBWReleased_flg = FALSE;
    VTQD_PBWLocked_flg = FALSE;
    VTQD_PBWUnlockTO_flg = FALSE;
    VTQD_PBWLockTO_flg = FALSE;
    state Initialize [commented out]
      en:
      VTQD_PBWUnlockTO_flg = FALSE;
      VTQD_PBWReleased_flg = FALSE;
      VTQD_PBWLocked_flg = FALSE;
    state PBWUnlock [commented out]
      en:
      VTQD_ParkRequest_flg = FALSE;
      (default) -> (junction 798) [commented out] : {
          | VTQD_PBWWaitTime_s = 0;
          | }
      PBWUnlock -> (junction 798) [commented out]
      (junction 798) -> (junction 799) [commented out] : [VINP_PBWMotorPos_enum == ENUM_PBWPOSITION_UNPARKED]
      (junction 798) -> (junction 800) [commented out] : {
          | VTQD_PBWWaitTime_s += task_time_s;
          | }
      (junction 799) -> (junction 804) [commented out] : {
          | VTQD_PBWReleased_flg = TRUE;
          | }
      (junction 800) -> (junction 801) [commented out] : [VTQD_PBWWaitTime_s >= KTQD_PBWTimeout_s]
      (junction 800) -> (junction 802) [commented out]
      (junction 801) -> (junction 803) [commented out] : {
          | VTQD_PBWUnlockTO_flg = TRUE;
          | }
      (junction 803) -> (junction 802) [commented out]
      (junction 804) -> (junction 803) [commented out]
    state PBWLock [commented out]
      en:
      VTQD_ParkRequest_flg = TRUE;
      (default) -> (junction 817) [commented out] : {
          | VTQD_PBWWaitTime_s = 0;
          | }
      (junction 817) -> (junction 816) [commented out] : [VINP_PBWMotorPos_enum == ENUM_PBWPOSITION_PARKED]
      PBWLock -> (junction 817) [commented out]
      (junction 816) -> (junction 822) [commented out] : {
          | VTQD_PBWLocked_flg = TRUE;
          | }
      (junction 817) -> (junction 818) [commented out] : {
          | VTQD_PBWWaitTime_s += task_time_s;
          | }
      (junction 818) -> (junction 819) [commented out] : [VTQD_PBWWaitTime_s >= KTQD_PBWTimeout_s]
      (junction 818) -> (junction 820) [commented out]
      (junction 819) -> (junction 821) [commented out] : {
          | VTQD_PBWLockTO_flg = TRUE;
          | }
      (junction 821) -> (junction 820) [commented out]
      (junction 822) -> (junction 821) [commented out]
    (default) -> PBW_Judgement.Initialize [commented out]
    PBW_Judgement.Initialize -> PBWUnlock [commented out] : [VTQD_GearShiftCMD_enum != ENUM_GEARSHIFTCMD_P]
    PBW_Judgement.Initialize -> PBWLock [commented out] : [VTQD_GearShiftCMD_enum == ENUM_GEARSHIFTCMD_P]
  state N
    en:
    VTQD_GearActualPosn_enum = ENUM_GEARACTUALPOSN_N;
    VTQD_ParkRequest_flg = FALSE;
    VTQD_EnterP_flg = FALSE;
    (default) -> (junction 753) : {
        | VTQD_RelockWaitTime_s = 0;
        | }
    (junction 753) -> (junction 754) [order 1] : %[!VTQD_PBWLockTO_flg]
    N -> (junction 753) [order 1]
    (junction 753) -> (junction 755) [order 2] : {
        | VTQD_RelockWaitTime_s += task_time_s;
        | }
    (junction 754) -> (junction 757) : {
        | VTQD_EnterP_flg = TRUE;
        | }
    (junction 755) -> (junction 756) [order 1] : [VTQD_RelockWaitTime_s >= KTQD_RelockWaitTime_s]
    (junction 755) -> (junction 760) [order 2]
    (junction 756) -> (junction 758) : {
        | VTQD_EnterP_flg = TRUE;
        | }
    (junction 758) -> (junction 760)
    (junction 757) -> (junction 758)
  state P
    en:
    VTQD_GearActualPosn_enum = ENUM_GEARACTUALPOSN_P;
    VTQD_ParkRequest_flg = TRUE;
    VTQD_ExitP_flg = FALSE;
    (default) -> (junction 867) : {
        | VTQD_ReunlockWaitTime_s = 0;
        | }
    P -> (junction 867) [order 1]
    (junction 867) -> (junction 868) [order 1] : %[!VTQD_PBWUnlockTO_flg]
    (junction 867) -> (junction 877) [order 2] : {
        | VTQD_ReunlockWaitTime_s += task_time_s;
        | }
    (junction 868) -> (junction 883) : {
        | VTQD_ExitP_flg = TRUE;
        | }
    (junction 877) -> (junction 880) [order 1] : [VTQD_ReunlockWaitTime_s >= KTQD_ReunlockWaitTime_s]
    (junction 877) -> (junction 871) [order 2]
    (junction 880) -> (junction 869) : {
        | VTQD_ExitP_flg = TRUE;
        | }
    (junction 869) -> (junction 871)
    (junction 883) -> (junction 869)
  state D
    en:
    VTQD_GearActualPosn_enum = ENUM_GEARACTUALPOSN_D;
    VTQD_ParkRequest_flg = FALSE;
  state R
    en:
    VTQD_GearActualPosn_enum = ENUM_GEARACTUALPOSN_R;
    VTQD_ParkRequest_flg = FALSE;
  (default) -> P : {
      |  VTQD_PBWLockTO_flg = FALSE;
      |  VTQD_PBWUnlockTO_flg = FALSE;
      | }
  N -> (junction 731) [order 2] : [VTQD_GearShiftCMD_enum == ENUM_GEARSHIFTCMD_R && VTQD_PwrStaAllowDR_flg &&...
      |  VTQD_TMRotateDirction_enum ~= ENUM_TMROTATEDIRECTACT_FORWARD &&...
      |  VTQD_BrkSwSta_flg]
      | %add20240710
  P -> N [order 1] : [(VTQD_GearShiftCMD_enum == ENUM_GEARSHIFTCMD_N &&...
      | VTQD_PwrStaAllowPN_flg && VTQD_BrkSwSta_flg && VTQD_ExitP_flg)&&...
      | !VTQD_ForceP_flg]
      | %add202400710
  (junction 731) -> (junction 733)
  (junction 749) -> N
  N -> P [order 3] : [(VTQD_GearShiftCMD_enum == ENUM_GEARSHIFTCMD_P && VTQD_PwrStaAllowPN_flg &&...
      |  VINP_VehSpd_kph <= KTQD_VehSpd2P_kph && VTQD_EnterP_flg) || VTQD_ForceP_flg ]
      | %add20240308
  (junction 747) -> (junction 749)
  D -> N [order 1] : [VTQD_GearShiftCMD_enum == ENUM_GEARSHIFTCMD_N ||...
      | !VTQD_PwrStaAllowDR_flg]
      | %20240710
  N -> D [order 1] : [VTQD_GearShiftCMD_enum == ENUM_GEARSHIFTCMD_D && VTQD_PwrStaAllowDR_flg &&...
      |  VTQD_TMRotateDirction_enum ~= ENUM_TMROTATEDIRECTACT_REVERSE]
      | %add20240710
  P -> D [order 2] : [VTQD_GearShiftCMD_enum == ENUM_GEARSHIFTCMD_D &&...
      | VTQD_PwrStaAllowDR_flg && VTQD_BrkSwSta_flg && VTQD_ExitP_flg &&...
      |  !VTQD_ForceP_flg]
      | %add20240710
  D -> P [order 2] : [(VTQD_GearShiftCMD_enum == ENUM_GEARSHIFTCMD_P && VTQD_PwrStaAllowPN_flg &&...
      |  VINP_VehSpd_kph <= KTQD_VehSpd2P_kph) || VTQD_ForceP_flg]
      | %add20240308
  R -> D [order 3] : [VTQD_GearShiftCMD_enum == ENUM_GEARSHIFTCMD_D && VTQD_PwrStaAllowDR_flg &&...
      |  VTQD_BrkSwSta_flg &&...
      |  VINP_VehSpd_kph <= KTQD_VehSpdRev_kph]
      | %add20240710
  D -> R [order 3] : [VTQD_GearShiftCMD_enum == ENUM_GEARSHIFTCMD_R && VTQD_PwrStaAllowDR_flg &&...
      |  VTQD_BrkSwSta_flg &&...
      | VINP_VehSpd_kph <= KTQD_VehSpdRev_kph]
      | %add20240710
  P -> R [order 3] : [VTQD_GearShiftCMD_enum == ENUM_GEARSHIFTCMD_R &&...
      | VTQD_PwrStaAllowDR_flg && VTQD_BrkSwSta_flg && VTQD_ExitP_flg && !VTQD_ForceP_flg]
      | %add20240710
  R -> (junction 747) [order 1] : [VTQD_GearShiftCMD_enum == ENUM_GEARSHIFTCMD_N ||...
      | !VTQD_PwrStaAllowDR_flg]
      | %add20240710
  (junction 733) -> R
  R -> P [order 2] : [(VTQD_GearShiftCMD_enum == ENUM_GEARSHIFTCMD_P && VTQD_PwrStaAllowPN_flg &&...
      |  VINP_VehSpd_kph <= KTQD_VehSpd2P_kph) || VTQD_ForceP_flg]
      | %add20240308
  data: task_time_s input; VTQD_BrkSwSta_flg input; VTQD_GearShiftCMD_enum input; VINP_VehSpd_kph input; VINP_PBWMotorPos_enum input; VTQD_PwrStaAllowDR_flg input; VTQD_PwrStaAllowPN_flg input; VTQD_TMRotateDirction_enum input; VTQD_GearActualPosn_enum output uint8; ENUM_GEARACTUALPOSN_N parameter; ENUM_GEARACTUALPOSN_D parameter; ENUM_GEARACTUALPOSN_R parameter; ENUM_GEARACTUALPOSN_P parameter; KTQD_VehSpd2P_kph input; VTQD_InitializeTime_s local single; ENUM_GEARACTUALPOSN_INVALID parameter; FALSE parameter; TRUE parameter; VTQD_ShiftInitialComplete_flg local boolean; ENUM_GEARSHIFTCMD_D parameter; ENUM_GEARSHIFTCMD_P parameter; ENUM_GEARSHIFTCMD_R parameter; ENUM_GEARSHIFTCMD_N parameter; KTQD_VehSpdRev_kph input; KTQD_ShiftInitialTime_s input; ENUM_PBWPOSITION_PARKED parameter; ENUM_PBWPOSITION_UNPARKED parameter; VTQD_PBWLockTO_flg output boolean; VTQD_PBWUnlockTO_flg output boolean; KTQD_PBWTimeout_s input; KTQD_RelockWaitTime_s input; KTQD_ReunlockWaitTime_s input; VTQD_ParkRequest_flg output boolean; VTQD_EnterP_flg local boolean; VTQD_ExitP_flg local boolean; VTQD_PBWLocked_flg local boolean; VTQD_PBWReleased_flg local boolean; VTQD_PBWWaitTime_s local single; VTQD_RelockWaitTime_s local single; VTQD_ReunlockWaitTime_s local single; ENUM_TMROTATEDIRECTACT_FORWARD parameter; ENUM_TMROTATEDIRECTACT_REVERSE parameter; VTQD_ForceP_flg input
